simulink model "nnn_cassie_sims"  (R2017b)
settings: Solver=VariableStepAuto  StartTime=0.0  StopTime=30
InitFcn:
  | PreFunctionss.PreParamss;
  | PreFunctionss.GaitData;
model workspace (MATLAB code in the model file):
  | PreFunctionss.BusInfoss
  | PreFunctionss.BusDataS
values from neighbouring files (symbols this model uses):
  s = min(s_unsat,1.05)    [ControllerS.m]
undefined symbols (not defined in the file or in its folder): fcut_velocity_joint, GaitLibrary, motorPositions, motorVelocities, pelvisPosition, pelvisVelocity, sampleTime, X, Y, Z
libraries: sm_lib x83, nesl_utility x17, ComponentLibrary x10, Contact_Forces_Lib x4, CassieLibrary x4, etargetslib x1, instrumentlib x1, simulink x1
(part 1 of 4)
settings Model: Creator=ls  LastModifiedBy=hanli
settings SolverCC: ZeroCrossControl=DisableAll
settings DataIOCC: SaveOutput=off  SignalLogging=off  DSMLogging=off  SaveTime=off
settings OptimizationCC: DefaultParameterBehavior=Inlined  UseFloatMulNetSlope=on  InlineInvariantSignals=on  EfficientFloat2IntCast=on  LifeSpan=inf  SimCompilerOptimization=on  AccelVerboseBuild=on
settings DebuggingCC: ReadBeforeWriteMsg=DisableAll  WriteAfterWriteMsg=DisableAll  WriteAfterReadMsg=DisableAll  ParameterUnderflowMsg=error  UniqueDataStoreMsg=error
settings ModelReferenceCC: EnableParallelModelReferenceBuilds=on  ModelReferenceNumInstancesAllowed=Zero  ModelReferenceMinAlgLoopOccurrences=on  PropagateSignalLabelsOutOfModel=off
settings SFSimCC: SimUserSources=vcom_casia_nnn_src.c pcom_casia_nnn_src.c p_toe_joint_right_src.c p_toe_joint_left_src.c p_RightToeFront_src.c p_RightToeBottom_src.c p_RightToeBack_src.c p_LeftToeFront_src.c p_LeftToeBottom_src.c p_LeftToeBack_src.c Jp_LeftToeBack_src.c Jp_RightToeBack_src.c Jp_toe_joint_left_src.c Jp_toe_joint_right_src.c
settings RTWCC: BuildConfiguration=Faster Runs  CheckMdlBeforeBuild=Warning
settings CodeAppCC: GenerateComments=off  SimulinkBlockComments=off
settings GRTTargetCC: MultiInstanceERTCode=on  CodeInterfacePackaging=Reusable function  SupportNonFinite=off  GenerateAllocFcn=on
settings ConfigComp: CovMetricSettings=dw  CovHtmlReporting=on  CovSaveSingleToWorkspaceVar=on
settings SimscapeCC: SimscapeNormalizeSystem=off
settings DiagnosticsConfigSet: SimMechanicsRigidlyBoundBlock=none

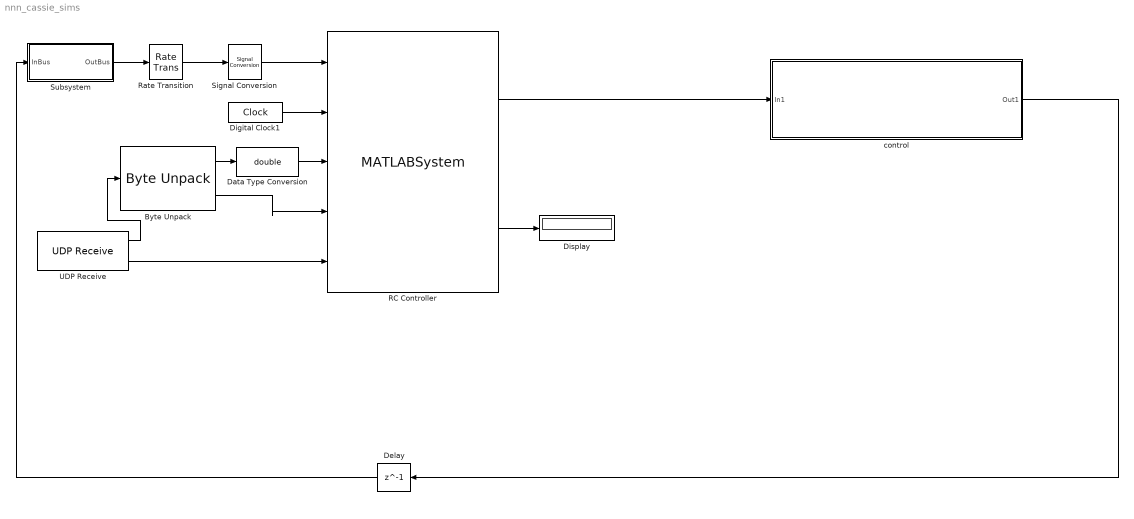
== system nnn_cassie_sims ==
  Byte Unpack : etargetslib/Byte Unpack  dimensions={1, [5,1]}  datatypes={'uint8','double'}  byteAlign=1
  Data Type Conversion : DataTypeConversion  OutDataTypeStr=double
  Delay : Delay  DelayLength=1  InitialCondition=0
  Digital Clock1 : DigitalClock  SampleTime=sampleTime
  Display : Display
  RC Controller : MATLABSystem  System=remote_controller  SimulateUsing=Code generation
      mask Type: remote_controller
      mask Display:
      | disp('remote_controller');
      | port_label('input',1,'cassieOut');
      | port_label('input',2,'t');
      | port_label('input',3,'sba');
      | port_label('input',4,'cmd');
      | port_label('input',5,'u_status');
      | port_label('output',1,'cassieOuts');
      | port_label('output',2,'rc_status');
  Rate Transition : RateTransition  Deterministic=off
  Signal Conversion : SignalConversion  ConversionOutput=Nonvirtual bus  OutDataTypeStr=Bus: CassieOutBus  OverrideOpt=off
  Subsystem : Subsystem
  UDP Receive : instrumentlib/UDP Receive  Host=192.168.3.4  Port=11223  LocalPort=11223  DataSize="[41   1]"  EnableBlockingMode=off  Timeout=10  SampleTime=0.0005  DataType=uint8  ByteOrder=BigEndian
      settings: SourceProductName=Instrument Control Toolbox
  control : Subsystem
  wires:
  RC Controller/1 -> control/1(In1)
  control/1(Out1) -> Delay/1
  Subsystem/1(OutBus) -> Rate Transition/1
  Signal Conversion/1 -> RC Controller/1
  Rate Transition/1 -> Signal Conversion/1
  Delay/1 -> Subsystem/1(InBus)
  Digital Clock1/1 -> RC Controller/2
  UDP Receive/1 -> Byte Unpack/1
  Byte Unpack/2 -> RC Controller/4
  UDP Receive/2 -> RC Controller/5
  Data Type Conversion/1 -> RC Controller/3
  Byte Unpack/1 -> Data Type Conversion/1
  RC Controller/2 -> Display/1

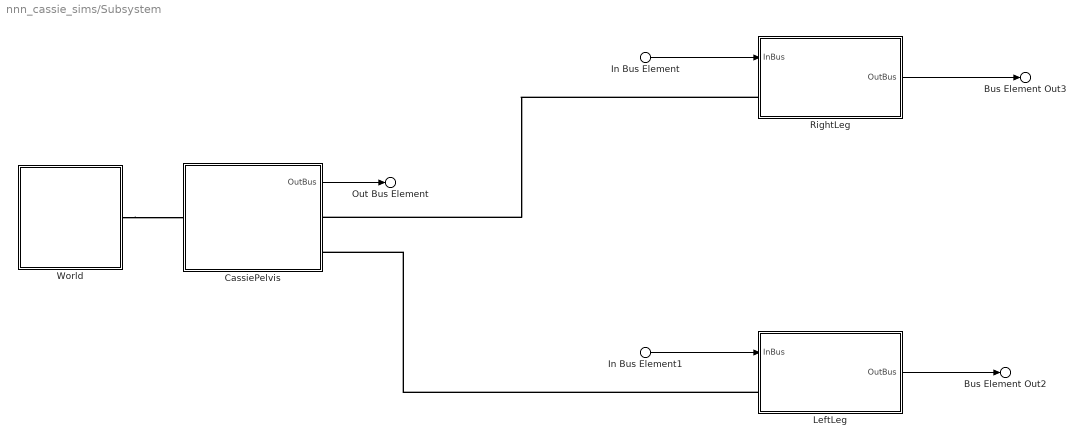
== system nnn_cassie_sims/Subsystem ==
  In Bus Element1 : Inport  PortName=InBus  Element=leftLeg
  In Bus Element : Inport  PortName=InBus  Element=rightLeg
  CassiePelvis : Subsystem
  LeftLeg : Subsystem
  RightLeg : Subsystem
  World : Subsystem  AncestorBlock=ComponentLibrary/Simulation/World
  Out Bus Element : Outport  PortName=OutBus  Element=pelvis
  Bus Element Out3 : Outport  PortName=OutBus  Element=rightLeg
  Bus Element Out2 : Outport  PortName=OutBus  Element=leftLeg
  wires:
  CassiePelvis/1(OutBus) -> Out Bus Element/1
  LeftLeg/1(OutBus) -> Bus Element Out2/1
  In Bus Element1/1 -> LeftLeg/1(InBus)
  In Bus Element/1 -> RightLeg/1(InBus)
  RightLeg/1(OutBus) -> Bus Element Out3/1
  connections:
  World/RConn1 -- CassiePelvis/LConn1
  LeftLeg/LConn1 -- CassiePelvis/RConn2
  RightLeg/LConn1 -- CassiePelvis/RConn1

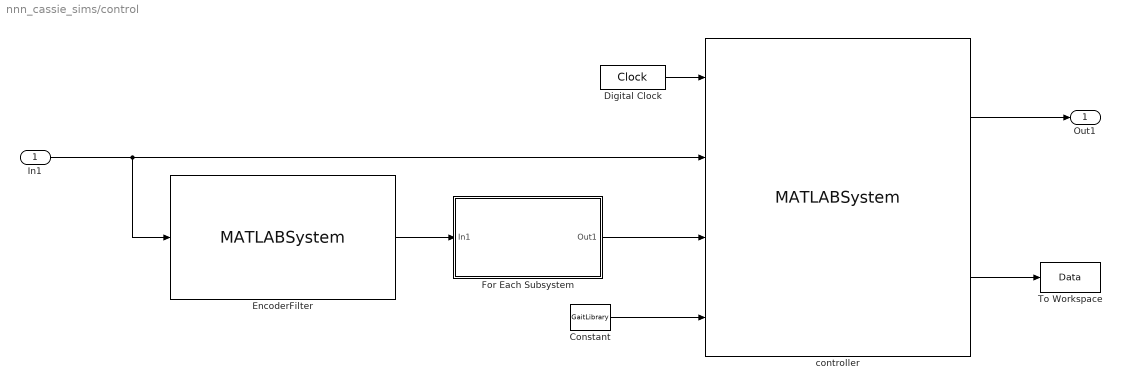
== system nnn_cassie_sims/control ==
  In1 : Inport
  Constant : Constant  Value=GaitLibrary  OutDataTypeStr=Bus: cassieGaitLibraryBus  LockScale=on
  Digital Clock : DigitalClock  SampleTime=sampleTime
  EncoderFilter : MATLABSystem  System=EncoderFilterS  SimulateUsing=Code generation
      mask Type: EncoderFilterS
      mask Display:
      | disp('EncoderFilterS');
      | port_label('input',1,'CassieOutputs');
      | port_label('output',1,'JointPosition');
  For Each Subsystem : Subsystem  TreatAsAtomicUnit=on
  To Workspace : ToWorkspace  VariableName=Data  SaveFormat=Timeseries  SampleTime=-1
  controller : MATLABSystem  System=ControllerS  Kp_toe_stand=c_Kp_toe_stand  Kd_toe_stand=c_Kd_toe_stand  Kp_lateral_stand=c_Kp_lateral_stand  Kd_lateral_stand=c_Kd_lateral_stand  Kp_abduction_stand=c_Kp_abduction_stand  Kd_abduction_stand=c_Kd_abduction_stand  Kp_thigh_stand=c_Kp_thigh_stand  Kd_thigh_stand=c_Kd_thigh_stand  Kp_knee_stand=c_Kp_knee_stand  Kd_knee_stand=c_Kd_knee_stand  Kp_rotation_stand=c_Kp_rotation_stand  Kd_rotation_stand=c_Kd_rotation_stand  joint_filter_choice=c_joint_filter_chocie  fil_para_x=c_fil_para_x  fil_para_y=c_fil_para_y  fil_para_2=c_fil_para_2  fil_para_3=c_fil_para_3  fil_para_4=c_fil_para_4  fil_para_5=c_fil_para_5  stance_thre_ub=c_stance_thre_ub  stance_thre_lb=c_stance_thre_lb  Kp_pitch=c_Kp_pitch  Kd_pitch=c_Kd_pitch  Kp_roll=c_Kp_roll  Kd_roll=c_Kd_roll  Kp_yaw=c_Kp_yaw  Kd_yaw=c_Kd_yaw  Kp_abduction=c_Kp_abduction  Kp_rotation=c_Kp_rotation  Kp_thigh=c_Kp_thigh  Kp_knee=c_Kp_knee  Kp_toe=c_Kp_toe  Kd_abduction=c_Kd_abduction  Kd_rotation=c_Kd_rotation  Kd_thigh=c_Kd_thigh  Kd_knee=c_Kd_knee  Kd_toe=c_Kd_toe  shift_time=c_shift_time  shift_distance=c_shift_distance  standing_switch_time=c_standing_switch_time  lateral_velocity_weight=c_lateral_velocity_weight  init_lateral_velocity=c_init_lateral_velocity  force_step_end_s=c_force_step_end_s  Kfs_p=c_Kfs_p  Kfl_p=c_Kfl_p  Kfs_d=c_Kfs_d  Kfl_d=c_Kfl_d  abduction_inward_gain=c_abduction_inward_gain  toe_tilt_angle=c_toe_tilt_angle  final_sw_abduction=c_final_sw_abduction  final_st_abduction=c_final_st_abduction  pre_final_sw_abduction=c_pre_final_sw_abduction  u_abduction_cp=c_u_abduction_cp  u_abduction_swing_cp=c_u_abduction_swing_cp  u_thigh_cp=c_u_thigh_cp  u_knee_cp=c_u_knee_cp  SimulateUsing=Code generation
      mask Type: ControllerS
      mask Display:
      | disp('ControllerS');
      | port_label('input',1,'t');
      | port_label('input',2,'cassie_data');
      | port_label('input',3,'encoder_fil');
      | port_label('input',4,'GaitLibrary');
      | port_label('output',1,'CasiaBBRInputs');
      | port_label('output',2,'log');
  Out1 : Outport
  wires:
  Digital Clock/1 -> controller/1
  EncoderFilter/1 -> For Each Subsystem/1(In1)
  controller/2 -> To Workspace/1
  In1/1 -> EncoderFilter/1, controller/2
  For Each Subsystem/1(Out1) -> controller/3
  controller/1 -> Out1/1
  Constant/1 -> controller/4

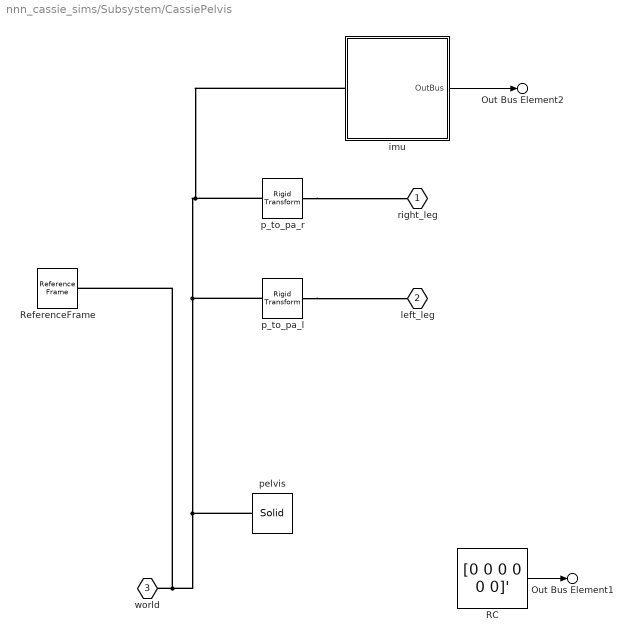
== system nnn_cassie_sims/Subsystem/CassiePelvis ==
  RC : Constant  Value=[0 0 0 0 0 0]'
  ReferenceFrame : sm_lib/Frames and Transforms/Reference Frame
  imu : Subsystem  AncestorBlock=ComponentLibrary/Simulation/VectorNav  mask{preRotationMatrix=[1, 0, 0; 0, 1, 0; 0, 0, 1], postRotationMatrix=[1, 0, 0; 0, 1, 0; 0, 0, 1]}
      mask prompts: preRotationMatrix "Pre Rotation Matrix:"; postRotationMatrix "Post Rotation Matrix"
      mask Display: image('VectorNav.png');
  p_to_pa_l : sm_lib/Frames and Transforms/Rigid Transform  TranslationMethod=Cartesian  TranslationStandardOffset=0  TranslationLengthUnit=m  TranslationStandardAxis=+Z  TranslationCartesianOffset=[0.018, 0.13451, -0.047805]  TranslationROffset=0  TranslationROffsetUnits=m  TranslationZOffset=0  TranslationZOffsetUnits=m  TranslationThetaOffset=0  TranslationThetaOffsetUnits=deg  RotationMethod=RotationMatrix  RotationAngleUnits=deg  RotationStandardAxis=+Z  RotationAngle=0.0  RotationArbitraryAxis=[0 0 1]  FollAlignAxisA=+X  BaseAlignAxisA=+Y  FollAlignAxisB=+Y  BaseAlignAxisB=+Z  RotationSequenceAxes=BaseAxes  RotationSequence=XYZ  RotationSequenceAngles=[0, 1.5708, 0]  RotationSequenceAnglesUnits=rad  RotationMatrix=[0 0 1; 0 1 0; -1 0 0]
  p_to_pa_r : sm_lib/Frames and Transforms/Rigid Transform  TranslationMethod=Cartesian  TranslationStandardOffset=0  TranslationLengthUnit=m  TranslationStandardAxis=+Z  TranslationCartesianOffset=[0.018, -0.13451, -0.047805]  TranslationROffset=0  TranslationROffsetUnits=m  TranslationZOffset=0  TranslationZOffsetUnits=m  TranslationThetaOffset=0  TranslationThetaOffsetUnits=deg  RotationMethod=RotationMatrix  RotationAngleUnits=deg  RotationStandardAxis=+Z  RotationAngle=0.0  RotationArbitraryAxis=[0 0 1]  FollAlignAxisA=+X  BaseAlignAxisA=+Y  FollAlignAxisB=+Y  BaseAlignAxisB=+Z  RotationSequenceAxes=BaseAxes  RotationSequence=XYZ  RotationSequenceAngles=[0, 1.5708, 0]  RotationSequenceAnglesUnits=rad  RotationMatrix=[0 0 1; 0 1 0;-1 0 0]
  pelvis : sm_lib/Body Elements/Solid  InertiaType=Custom  Mass=6.56964969274137  MassUnits=kg  CenterOfMass=[0.0295583628182488, 3.89626767704742e-05, -0.0155783424997369]  CenterOfMassUnits=m  MomentsOfInertia=[0.0235604863264443, 0.014455865873678, 0.010763598299641]  MomentsOfInertiaUnits=kg*m^2  ProductsOfInertia=[-6.61650817705804e-07, 7.97597097465651e-06, -2.84451907912671e-06]  ProductsOfInertiaUnits=kg*m^2  DensityBased=on  Density=1000  DensityUnits=kg/m^3  DoExposeReferenceFrame=on  SerializedFrames=<Frames/>  GraphicType=FromGeometry  MarkerShape=Sphere  MarkerSize=10  GraphicVisPropType=SimpleVisualProperties  GraphicDiffuseColor=[0.898039215686275, 0.917647058823529, 0.929411764705882]  GraphicSpecularColor=[0.5 0.5 0.5 1.0]  GraphicAmbientColor=[0.15 0.15 0.15 1.0]  GraphicEmissiveColor=[0.0 0.0 0.0 1.0]  GraphicShininess=75  GraphicOpacity=1  GeometryShape=FromFile  RectangleSize=[1 1]  RectangleSizeUnits=m  BrickDimensions=[1 1 1]  BrickDimensionUnits=m  CylinderRadius=1  CylinderRadiusUnits=m  CylinderLength=1  CylinderLengthUnits=m  SphereRadius=1  SphereRadiusUnits=m  EllipsoidRadii=[1 1 1]  EllipsoidRadiiUnits=m  ExtrusionCrossSection=[1 1; -1 1; -1 -1; 1 -1]  ExtrusionCrossSectionUnits=m  ExtrusionLength=1  ExtrusionLengthUnits=m  PolygonNumSides=3  PolygonOuterRadius=1  PolygonOuterRadiusUnits=m  ExtGeomFileType=STL  ExtGeomFileName=meshes/pelvis.STL  ExtGeomFileUnits=m  RevolutionCrossSection=[1 1; 1 -1; 2 -1; 2 1]  RevolutionCrossSectionUnits=m  RevolutionExtent=Full  RevolutionAngle=180  RevolutionAngleUnits=deg
  right_leg : PMIOPort  Port=1  Side=Right
  left_leg : PMIOPort  Port=2  Side=Right
  world : PMIOPort  Port=3  Side=Left
  Out Bus Element1 : Outport  PortName=OutBus  Element=RC
  Out Bus Element2 : Outport  PortName=OutBus  Element=IMU
  wires:
  RC/1 -> Out Bus Element1/1
  imu/1(OutBus) -> Out Bus Element2/1
  connections:
  imu/LConn1 -- p_to_pa_r/LConn1 -- p_to_pa_l/LConn1 -- pelvis/RConn1 -- ReferenceFrame/RConn1 -- world/RConn1
  p_to_pa_r/RConn1 -- right_leg/RConn1
  p_to_pa_l/RConn1 -- left_leg/RConn1
